simulink model "DblLaneChange_nn"  (R2018a)
settings: Solver=VariableStepAuto  StartTime=0.0  StopTime=10.0  RelTol=1e-3
libraries: neural x42
(part 2 of 2)

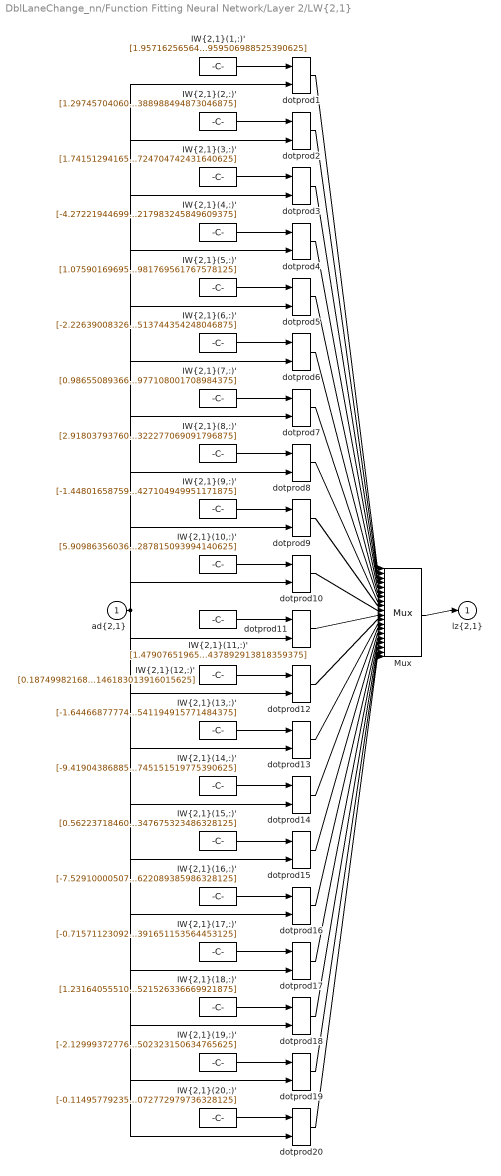
== system DblLaneChange_nn/Function Fitting Neural Network/Layer 2/LW{2,1} ==
  "ad{2,1}" : Inport  PortDimensions=15
      mask Display: e = 0.06;c1 = [120 230 180]/255;c2 = ([120 230 180]+0)/(256+128);c3 = ([120 230 180]+128)/(256+128);patch([0 1 1 0],[0 0 1 1],c1);patch([0 1 1 1-e 1-e 0+e],[0 0 1 1-e 0+e 0+e],c2);patch([0 0 1 1-e 0+e 0+e],[0 1 1 1-e 1-e 0+e],c3);plot([0 1 1 0 0],[0 0 1 1 0]);
  "IW{2,1}(1,:)'" : Constant  Value=[1.9571625656470332810243917265324853360652923583984375;3.8878561459758547158571673207916319370269775390625;2.015104111831793165521276023355312645435333251953125;-3.3420079123150543409792589955031871795654296875;-0.250819509672329743477092733883182518184185028076171875;0.6739952161544857656139129176153801381587982177734375;-1.3339737299760254796154868017765693366527557373046875;0.272342183832987583258500308147631585597991943359375;-0.04635129880112805189629199276168947108089923858642578125;-3.00793871482913033332806662656366825103759765625;0.251349256199478843232242297744960524141788482666015625;0.1750736907436108158453436089985189028084278106689453125;2.48237885981700845405839572777040302753448486328125;0.281589867390764025945060211597592569887638092041015625;-0.5513138093502016889857486603432334959506988525390625]
      mask Display: e = 0.06;c1 = [120 150 230]/255;c2 = ([120 150 230]+0)/383;c3 = ([120 150 230]+128)/383;patch([0 1 1 0],[0 0 1 1],c1);patch([0 1 1 1-e 1-e 0+e],[0 0 1 1-e 0+e 0+e],c2);patch([0 0 1 1-e 0+e 0+e],[0 1 1 1-e 1-e 0+e],c3);plot([0 1 1 0 0],[0 0 1 1 0]);disp('weights');
  "IW{2,1}(10,:)'" : Constant  Value=[5.90986356036200621844045599573291838169097900390625;-2.137684664328248107523222643067128956317901611328125;-3.226180872466682725274722542962990701198577880859375;2.398560219815558891554019282921217381954193115234375;-0.351261492817215692507915036912891082465648651123046875;1.756271886281308258759281670791096985340118408203125;-0.32097773012757924160354150444618426263332366943359375;2.0890044930821982660518187913112342357635498046875;-1.55820878601203549607134846155531704425811767578125;-0.399566441545824380110474294269806705415248870849609375;0.12749773005068154585472939288592897355556488037109375;0.0480334247417505133537218853234662674367427825927734375;0.0992931501305693575698541053498047403991222381591796875;-0.60598205258813242490845141219324432313442230224609375;-1.1258930863377900610799997593858279287815093994140625]
      mask Display: e = 0.06;c1 = [120 150 230]/255;c2 = ([120 150 230]+0)/383;c3 = ([120 150 230]+128)/383;patch([0 1 1 0],[0 0 1 1],c1);patch([0 1 1 1-e 1-e 0+e],[0 0 1 1-e 0+e 0+e],c2);patch([0 0 1 1-e 0+e 0+e],[0 1 1 1-e 1-e 0+e],c3);plot([0 1 1 0 0],[0 0 1 1 0]);disp('weights');
  "IW{2,1}(11,:)'" : Constant  Value=[1.479076519650180276954642977216280996799468994140625;-1.8264341661270770966751797459437511861324310302734375;-9.6450188180864966369654212030582129955291748046875;3.30452725241774469822075843694619834423065185546875;-1.062855642218289542455522678210400044918060302734375;2.373360663004012049981383825070224702358245849609375;-0.246008815611256370647907942839083261787891387939453125;-2.130860279171088667027333940495736896991729736328125;-2.00602923066542526697730863816104829311370849609375;-0.872186134418087011255238394369371235370635986328125;-6.687297405909703229553997516632080078125;1.364795272975333428888689013547264039516448974609375;-0.47158321560510074732519569806754589080810546875;-2.933715231286582625358505538315512239933013916015625;0.231501625263715649083451353362761437892913818359375]
      mask Display: e = 0.06;c1 = [120 150 230]/255;c2 = ([120 150 230]+0)/383;c3 = ([120 150 230]+128)/383;patch([0 1 1 0],[0 0 1 1],c1);patch([0 1 1 1-e 1-e 0+e],[0 0 1 1-e 0+e 0+e],c2);patch([0 0 1 1-e 0+e 0+e],[0 1 1 1-e 1-e 0+e],c3);plot([0 1 1 0 0],[0 0 1 1 0]);disp('weights');
  "IW{2,1}(12,:)'" : Constant  Value=[0.18749982168050538522408032804378308355808258056640625;-2.4186038350858876100346606108359992504119873046875;-0.54761726970257684765641670310287736356258392333984375;3.651368967093746586982661028741858899593353271484375;-0.70468135689368216478811746128485538065433502197265625;1.000020555024070834093663506791926920413970947265625;0.5891913103732548950830505418707616627216339111328125;4.00129895607543772939607151784002780914306640625;-0.460439945014462781447406314327963627874851226806640625;-0.6516061444199390262355109371128492057323455810546875;-0.2617198429841096629644425775040872395038604736328125;-0.8055231764580004227838117003557272255420684814453125;0.84533215292148700115149040357209742069244384765625;1.7135058705183412453010305398493073880672454833984375;0.214677382943929073721989198020310141146183013916015625]
      mask Display: e = 0.06;c1 = [120 150 230]/255;c2 = ([120 150 230]+0)/383;c3 = ([120 150 230]+128)/383;patch([0 1 1 0],[0 0 1 1],c1);patch([0 1 1 1-e 1-e 0+e],[0 0 1 1-e 0+e 0+e],c2);patch([0 0 1 1-e 0+e 0+e],[0 1 1 1-e 1-e 0+e],c3);plot([0 1 1 0 0],[0 0 1 1 0]);disp('weights');
  "IW{2,1}(13,:)'" : Constant  Value=[-1.6446687777437969391058913970482535660266876220703125;1.0892551228031204235691120629780925810337066650390625;-0.007684977593027149909976625252738813287578523159027099609375;1.86688177259719623179989866912364959716796875;-6.7794873490613216659994577639736235141754150390625;-0.418152455463235706023539250963949598371982574462890625;3.51712271643014862121390251559205353260040283203125;2.65031843964746460784454029635526239871978759765625;-5.3869854890003079361804338986985385417938232421875;-0.356673648884901439704009362685610540211200714111328125;-0.2295944669061752152483535382998525165021419525146484375;3.041459947956777210009704504045657813549041748046875;-1.628179163118948391542062381631694734096527099609375;-4.4714054694712874749029651866294443607330322265625;-2.741411485446989981795695712207816541194915771484375]
      mask Display: e = 0.06;c1 = [120 150 230]/255;c2 = ([120 150 230]+0)/383;c3 = ([120 150 230]+128)/383;patch([0 1 1 0],[0 0 1 1],c1);patch([0 1 1 1-e 1-e 0+e],[0 0 1 1-e 0+e 0+e],c2);patch([0 0 1 1-e 0+e 0+e],[0 1 1 1-e 1-e 0+e],c3);plot([0 1 1 0 0],[0 0 1 1 0]);disp('weights');
  "IW{2,1}(14,:)'" : Constant  Value=[-9.419043868851968426270104828290641307830810546875;2.114542513786489497107368151773698627948760986328125;6.6725367883884754149903528741560876369476318359375;2.461496243771723602122847296413965523242950439453125;2.012042505986927576344669432728551328182220458984375;-0.072474795090835986144384150975383818149566650390625;1.400146161122375332297451677732169628143310546875;-9.1458682032511955384279644931666553020477294921875;1.98598101723450337630083595286123454570770263671875;-4.45193123880581342888262952328659594058990478515625;2.451062197202027892473097381298430263996124267578125;-1.73850853038267150196816146490164101123809814453125;-2.06427192595482011938656796701252460479736328125;0.340728899158648401712667919127852655947208404541015625;0.67217341264327468142170118881040252745151519775390625]
      mask Display: e = 0.06;c1 = [120 150 230]/255;c2 = ([120 150 230]+0)/383;c3 = ([120 150 230]+128)/383;patch([0 1 1 0],[0 0 1 1],c1);patch([0 1 1 1-e 1-e 0+e],[0 0 1 1-e 0+e 0+e],c2);patch([0 0 1 1-e 0+e 0+e],[0 1 1 1-e 1-e 0+e],c3);plot([0 1 1 0 0],[0 0 1 1 0]);disp('weights');
  "IW{2,1}(15,:)'" : Constant  Value=[0.562237184609895468412332775187678635120391845703125;-0.9456920295664283937497884835465811192989349365234375;-0.6311954154726482357773420517332851886749267578125;3.275377370304279001089753364794887602329254150390625;0.329026190777529148334679121035151183605194091796875;-0.380998484745070420398604937872732989490032196044921875;-0.80017096636857443225920860641053877770900726318359375;1.73199083915180285231372181442566215991973876953125;-0.2276919016580762067381016322542564012110233306884765625;0.437211733838442084820741229123086668550968170166015625;-0.305821512121914995674387682811357080936431884765625;-1.38121314321437527183888960280455648899078369140625;0.844141753276321793464376241900026798248291015625;-3.458095739856301253922765681636519730091094970703125;1.2818508895183697848807469199527986347675323486328125]
      mask Display: e = 0.06;c1 = [120 150 230]/255;c2 = ([120 150 230]+0)/383;c3 = ([120 150 230]+128)/383;patch([0 1 1 0],[0 0 1 1],c1);patch([0 1 1 1-e 1-e 0+e],[0 0 1 1-e 0+e 0+e],c2);patch([0 0 1 1-e 0+e 0+e],[0 1 1 1-e 1-e 0+e],c3);plot([0 1 1 0 0],[0 0 1 1 0]);disp('weights');
  "IW{2,1}(16,:)'" : Constant  Value=[-7.52910000507232357591647087247110903263092041015625;2.34534452763346923376275299233384430408477783203125;2.634914709341771743567051089485175907611846923828125;-4.0266144720965275638491220888681709766387939453125;0.10282036662459941023239906598973902873694896697998046875;-1.3053476659419194216837922795093618333339691162109375;1.05964548882387976647123650764115154743194580078125;-2.941417987553542001677442385698668658733367919921875;0.82654152921551860000448641585535369813442230224609375;-0.2530410430159644175063249349477700889110565185546875;-0.1848911532609083530065419154198025353252887725830078125;6.47931547167705002010507087106816470623016357421875;-0.3942440277240584212137264330522157251834869384765625;4.01703752952216408544927617185749113559722900390625;1.886129375602820790192026834120042622089385986328125]
      mask Display: e = 0.06;c1 = [120 150 230]/255;c2 = ([120 150 230]+0)/383;c3 = ([120 150 230]+128)/383;patch([0 1 1 0],[0 0 1 1],c1);patch([0 1 1 1-e 1-e 0+e],[0 0 1 1-e 0+e 0+e],c2);patch([0 0 1 1-e 0+e 0+e],[0 1 1 1-e 1-e 0+e],c3);plot([0 1 1 0 0],[0 0 1 1 0]);disp('weights');
  "IW{2,1}(17,:)'" : Constant  Value=[-0.71571123092296196066541824620799161493778228759765625;-0.92777937570890145480007049627602100372314453125;10.8447708602443899650324965477921068668365478515625;1.4015710214659271581894017799641005694866180419921875;-0.10900237728617911958650665837922133505344390869140625;-3.064976767817614966560313405352644622325897216796875;1.3560856151338160913155661546625196933746337890625;0.88919198881820282753807305198279209434986114501953125;-0.76945576277128691078388555979472585022449493408203125;-4.0863512374290440476443109218962490558624267578125;3.79150612913527407243918787571601569652557373046875;1.2389275360579159457330433724564500153064727783203125;-3.55580501974170903878302851808257400989532470703125;-5.18367612230348751012343200272880494594573974609375;-2.193181481708041946632192775723524391651153564453125]
      mask Display: e = 0.06;c1 = [120 150 230]/255;c2 = ([120 150 230]+0)/383;c3 = ([120 150 230]+128)/383;patch([0 1 1 0],[0 0 1 1],c1);patch([0 1 1 1-e 1-e 0+e],[0 0 1 1-e 0+e 0+e],c2);patch([0 0 1 1-e 0+e 0+e],[0 1 1 1-e 1-e 0+e],c3);plot([0 1 1 0 0],[0 0 1 1 0]);disp('weights');
  "IW{2,1}(18,:)'" : Constant  Value=[1.2316405551040798815876087246579118072986602783203125;-2.102966577787353852357910000137053430080413818359375;2.058306439730734016535507180378772318363189697265625;1.5042854125219804473090334795415401458740234375;0.07703822108708051341618983087755623273551464080810546875;-1.449657194903263945917615274083800613880157470703125;2.148337007307501433928109690896235406398773193359375;-2.710709509179739740147851989604532718658447265625;0.60574839965657900631157417592476122081279754638671875;0.65562455406318942419119366604718379676342010498046875;-1.473787306106492334123458931571803987026214599609375;0.421496584121772766007296695534023456275463104248046875;-0.60631975751951083797308683642768301069736480712890625;-5.44685251089520594547366272308863699436187744140625;0.2398404687163100401647852777387015521526336669921875]
      mask Display: e = 0.06;c1 = [120 150 230]/255;c2 = ([120 150 230]+0)/383;c3 = ([120 150 230]+128)/383;patch([0 1 1 0],[0 0 1 1],c1);patch([0 1 1 1-e 1-e 0+e],[0 0 1 1-e 0+e 0+e],c2);patch([0 0 1 1-e 0+e 0+e],[0 1 1 1-e 1-e 0+e],c3);plot([0 1 1 0 0],[0 0 1 1 0]);disp('weights');
  "IW{2,1}(19,:)'" : Constant  Value=[-2.129993727764210031949687618180178105831146240234375;-1.1272107118748539988928314414806663990020751953125;-0.69156568999726408808470523581490851938724517822265625;0.73787856477719693248928933826391585171222686767578125;2.049753693423387534977564428118057548999786376953125;-3.34020954313206974717331831925548613071441650390625;3.015120023433614182550854820874519646167755126953125;-0.8669712765240202845262729169917292892932891845703125;-7.0815027415871920624113045050762593746185302734375;-4.7342133957354004536455249763093888759613037109375;-1.699728451389623362643988002673722803592681884765625;0.4915630144269445001015128582366742193698883056640625;0.663091540309036275857579312287271022796630859375;2.44407792172628379745447091409005224704742431640625;-0.0389738779121663603266512154732481576502323150634765625]
      mask Display: e = 0.06;c1 = [120 150 230]/255;c2 = ([120 150 230]+0)/383;c3 = ([120 150 230]+128)/383;patch([0 1 1 0],[0 0 1 1],c1);patch([0 1 1 1-e 1-e 0+e],[0 0 1 1-e 0+e 0+e],c2);patch([0 0 1 1-e 0+e 0+e],[0 1 1 1-e 1-e 0+e],c3);plot([0 1 1 0 0],[0 0 1 1 0]);disp('weights');
  "IW{2,1}(2,:)'" : Constant  Value=[1.2974570406068279826428124579251743853092193603515625;0.125214635833320098168286449435981921851634979248046875;1.311851249355715509636866045184433460235595703125;0.79447946068844255140817267601960338652133941650390625;2.814888454915816407009288013796322047710418701171875;-0.65002613849646484478483898783451877534389495849609375;0.31816623644248964719594141570269130170345306396484375;-4.21939598665019133250098093412816524505615234375;-1.2418665807473938667016000181320123374462127685546875;0.90699287127850503065218390474910847842693328857421875;-0.73688571392916613067569642225862480700016021728515625;-3.933466164463143233120945296832360327243804931640625;-1.0353306206281096546462094920570962131023406982421875;1.1599716225973069061438991411705501377582550048828125;0.78680595520741558601685028406791388988494873046875]
      mask Display: e = 0.06;c1 = [120 150 230]/255;c2 = ([120 150 230]+0)/383;c3 = ([120 150 230]+128)/383;patch([0 1 1 0],[0 0 1 1],c1);patch([0 1 1 1-e 1-e 0+e],[0 0 1 1-e 0+e 0+e],c2);patch([0 0 1 1-e 0+e 0+e],[0 1 1 1-e 1-e 0+e],c3);plot([0 1 1 0 0],[0 0 1 1 0]);disp('weights');
  "IW{2,1}(20,:)'" : Constant  Value=[-0.1149577923562907499910323849690030328929424285888671875;3.49330095989750599727585722575895488262176513671875;2.19885314886025273750647102133370935916900634765625;-0.2651349581561339707747038119123317301273345947265625;1.13861957041805705870274323388002812862396240234375;0.8131303347112022184006718816817738115787506103515625;-0.9470707754184870541536156451911665499210357666015625;-2.198780912367476414459588340832851827144622802734375;-1.294167608085416087959629294346086680889129638671875;1.2105212187917084865063088727765716612339019775390625;-1.0764523265034167121001473788055591285228729248046875;-2.26989440626234095788049671682529151439666748046875;0.037344458215924518362793804726607049815356731414794921875;0.477151102120123737915236006301711313426494598388671875;0.355409142713680126224318200911511667072772979736328125]
      mask Display: e = 0.06;c1 = [120 150 230]/255;c2 = ([120 150 230]+0)/383;c3 = ([120 150 230]+128)/383;patch([0 1 1 0],[0 0 1 1],c1);patch([0 1 1 1-e 1-e 0+e],[0 0 1 1-e 0+e 0+e],c2);patch([0 0 1 1-e 0+e 0+e],[0 1 1 1-e 1-e 0+e],c3);plot([0 1 1 0 0],[0 0 1 1 0]);disp('weights');
  "IW{2,1}(3,:)'" : Constant  Value=[1.7415129416524244287955980325932614505290985107421875;4.60958769398082690571527564316056668758392333984375;1.853953325328213441736124877934344112873077392578125;-2.29169405563924488689053760026581585407257080078125;0.64410752453107156245692976881400682032108306884765625;-0.420812285627358395601049778633750975131988525390625;-0.1909525372905495899100714041196624748408794403076171875;-0.784172476643829607922953073284588754177093505859375;2.125282454412551036426748396479524672031402587890625;0.1907080131010278345460307036773883737623691558837890625;0.109625387283181108255547542285057716071605682373046875;-3.505620102081777655911309921066276729106903076171875;-0.03136599554879802853601944434558390639722347259521484375;-2.232858007504352482186504857963882386684417724609375;-0.47777926155416994280500375680276192724704742431640625]
      mask Display: e = 0.06;c1 = [120 150 230]/255;c2 = ([120 150 230]+0)/383;c3 = ([120 150 230]+128)/383;patch([0 1 1 0],[0 0 1 1],c1);patch([0 1 1 1-e 1-e 0+e],[0 0 1 1-e 0+e 0+e],c2);patch([0 0 1 1-e 0+e 0+e],[0 1 1 1-e 1-e 0+e],c3);plot([0 1 1 0 0],[0 0 1 1 0]);disp('weights');
  "IW{2,1}(4,:)'" : Constant  Value=[-4.2722194469990757426103300531394779682159423828125;12.1359268792165782002712148823775351047515869140625;25.62472900977618195383911370299756526947021484375;2.7555733226685266146205322002060711383819580078125;3.490286334781497412649287070962600409984588623046875;-0.10529579464098215435541305851074866950511932373046875;-4.142639466636097722584963776171207427978515625;-2.08334429948006327748544208589009940624237060546875;6.00228296822584894698593416251242160797119140625;-2.08162749754345810515587800182402133941650390625;16.386586981025402565137483179569244384765625;-2.183350057131614452288204120122827589511871337890625;-9.718174177731981444594566710293292999267578125;0.053049440768477840180139537551440298557281494140625;-1.3102285593647200467870561624295078217983245849609375]
      mask Display: e = 0.06;c1 = [120 150 230]/255;c2 = ([120 150 230]+0)/383;c3 = ([120 150 230]+128)/383;patch([0 1 1 0],[0 0 1 1],c1);patch([0 1 1 1-e 1-e 0+e],[0 0 1 1-e 0+e 0+e],c2);patch([0 0 1 1-e 0+e 0+e],[0 1 1 1-e 1-e 0+e],c3);plot([0 1 1 0 0],[0 0 1 1 0]);disp('weights');
  "IW{2,1}(5,:)'" : Constant  Value=[1.075901696950349872849983512423932552337646484375;-0.85654332659910126235303096109419129788875579833984375;2.3929012059066661066708547878079116344451904296875;-2.3067434710526750762937808758579194545745849609375;-2.510749704465401688224801546311937272548675537109375;3.32161347428343400878247848595492541790008544921875;-1.175453029695316065073029676568694412708282470703125;-1.290711021437697780811504344455897808074951171875;0.945242250920026005900353993638418614864349365234375;4.1259010747603550584017284563742578029632568359375;-3.4282086004042948701453497051261365413665771484375;-1.49349992078351068158781345118768513202667236328125;1.9574683298787702856458281530649401247501373291015625;0.74543647882154961958889316520071588456630706787109375;1.80109180790346545819602397386915981769561767578125]
      mask Display: e = 0.06;c1 = [120 150 230]/255;c2 = ([120 150 230]+0)/383;c3 = ([120 150 230]+128)/383;patch([0 1 1 0],[0 0 1 1],c1);patch([0 1 1 1-e 1-e 0+e],[0 0 1 1-e 0+e 0+e],c2);patch([0 0 1 1-e 0+e 0+e],[0 1 1 1-e 1-e 0+e],c3);plot([0 1 1 0 0],[0 0 1 1 0]);disp('weights');
  "IW{2,1}(6,:)'" : Constant  Value=[-2.2263900832626379866496790782548487186431884765625;1.13140963270349370617395834415219724178314208984375;-1.1152718875630813766264282094198279082775115966796875;2.9638683900000462045909443986602127552032470703125;-0.119020542071015811291800901017268188297748565673828125;0.89580900077017833194048535006004385650157928466796875;0.89086444994895785942645716204424388706684112548828125;2.55474733870291981219224908272735774517059326171875;0.2169307183781970793656768137225299142301082611083984375;-1.0705850496691204920551854229415766894817352294921875;-0.2086614854452577827448322977943462319672107696533203125;3.9627646343637454862118829623796045780181884765625;1.2081351444333849887158294222899712622165679931640625;3.595934259547820754931990450131706893444061279296875;0.69768729317174216220109883579425513744354248046875]
      mask Display: e = 0.06;c1 = [120 150 230]/255;c2 = ([120 150 230]+0)/383;c3 = ([120 150 230]+128)/383;patch([0 1 1 0],[0 0 1 1],c1);patch([0 1 1 1-e 1-e 0+e],[0 0 1 1-e 0+e 0+e],c2);patch([0 0 1 1-e 0+e 0+e],[0 1 1 1-e 1-e 0+e],c3);plot([0 1 1 0 0],[0 0 1 1 0]);disp('weights');
  "IW{2,1}(7,:)'" : Constant  Value=[0.98655089366556480978687204697052948176860809326171875;2.1074232656800422347487256047315895557403564453125;-0.58570887409710092885717358512920327484607696533203125;0.48233336801888448963637756605749018490314483642578125;0.09963593409410780032953169893517042510211467742919921875;-0.46646130605211599817749856811133213341236114501953125;0.5093470115656264507464356938726268708705902099609375;0.794409715381384717858281874214299023151397705078125;1.988294947404373846921998847392387688159942626953125;-0.002675882203754468245671116477524265064857900142669677734375;-0.372645169229664563470549865087377838790416717529296875;-0.465779993386511048658604750016820617020130157470703125;0.5158318737046130308954161591827869415283203125;0.320477121396944786280158723457134328782558441162109375;0.11922148986793366931546955811427324078977108001708984375]
      mask Display: e = 0.06;c1 = [120 150 230]/255;c2 = ([120 150 230]+0)/383;c3 = ([120 150 230]+128)/383;patch([0 1 1 0],[0 0 1 1],c1);patch([0 1 1 1-e 1-e 0+e],[0 0 1 1-e 0+e 0+e],c2);patch([0 0 1 1-e 0+e 0+e],[0 1 1 1-e 1-e 0+e],c3);plot([0 1 1 0 0],[0 0 1 1 0]);disp('weights');
  "IW{2,1}(8,:)'" : Constant  Value=[2.918037937604385234635628876276314258575439453125;0.94424412902173404660288724699057638645172119140625;-0.2308796501149148749920669843049836345016956329345703125;-0.5007912878569114045745891417027451097965240478515625;7.38580232235594547063328718650154769420623779296875;1.148002415199903314402263276861049234867095947265625;-2.501848844515395686727288193651475012302398681640625;-1.0255996771174886728061892426921986043453216552734375;2.4956843839866085232870318577624857425689697265625;-1.8420465154428089515903366191196255385875701904296875;-0.5092823515801596645502513638348318636417388916015625;-1.5218477171204740638899011173634789884090423583984375;-0.6844739356845443989385557870264165103435516357421875;2.099767731690322047910512992530129849910736083984375;3.210608297261831278746058160322718322277069091796875]
      mask Display: e = 0.06;c1 = [120 150 230]/255;c2 = ([120 150 230]+0)/383;c3 = ([120 150 230]+128)/383;patch([0 1 1 0],[0 0 1 1],c1);patch([0 1 1 1-e 1-e 0+e],[0 0 1 1-e 0+e 0+e],c2);patch([0 0 1 1-e 0+e 0+e],[0 1 1 1-e 1-e 0+e],c3);plot([0 1 1 0 0],[0 0 1 1 0]);disp('weights');
  "IW{2,1}(9,:)'" : Constant  Value=[-1.4480165875975588019031192743568681180477142333984375;-3.23195010974846841378393946797586977481842041015625;-1.7682767350317025734085518706706352531909942626953125;2.702804363845552781953074372722767293453216552734375;-1.9772495347968772616553678744821809232234954833984375;2.048857644404706856988696017651818692684173583984375;1.01523318616815938497666138573549687862396240234375;-3.83537556144572366889633485698141157627105712890625;-0.4756332520795110152533879954717122018337249755859375;1.7277037976748832459605864642071537673473358154296875;0.10589567856046207261488945050587062723934650421142578125;2.186685152170862789233751755091361701488494873046875;-1.5394951106473524493623017406207509338855743408203125;-0.113300141138904797433184512556181289255619049072265625;-0.384121670028321815504313008204917423427104949951171875]
      mask Display: e = 0.06;c1 = [120 150 230]/255;c2 = ([120 150 230]+0)/383;c3 = ([120 150 230]+128)/383;patch([0 1 1 0],[0 0 1 1],c1);patch([0 1 1 1-e 1-e 0+e],[0 0 1 1-e 0+e 0+e],c2);patch([0 0 1 1-e 0+e 0+e],[0 1 1 1-e 1-e 0+e],c3);plot([0 1 1 0 0],[0 0 1 1 0]);disp('weights');
  Mux : Mux  Inputs=20
      mask Display: e = 0.06;c1 = [120 150 230]/255;c2 = ([120 150 230]+0)/383;c3 = ([120 150 230]+128)/383;patch([0 1 1 0],[0 0 1 1],c1);patch([0 1 1 1-e 1-e 0+e],[0 0 1 1-e 0+e 0+e],c2);patch([0 0 1 1-e 0+e 0+e],[0 1 1 1-e 1-e 0+e],c3);plot([0 1 1 0 0],[0 0 1 1 0]);disp('Mux');
  dotprod{1..20} (20 alike) : neural/Weight Functions/dotprod
  "lz{2,1}" : Outport
      mask Display: e = 0.06;c1 = [120 230 180]/255;c2 = ([120 230 180]+0)/(256+128);c3 = ([120 230 180]+128)/(256+128);patch([0 1 1 0],[0 0 1 1],c1);patch([0 1 1 1-e 1-e 0+e],[0 0 1 1-e 0+e 0+e],c2);patch([0 0 1 1-e 0+e 0+e],[0 1 1 1-e 1-e 0+e],c3);plot([0 1 1 0 0],[0 0 1 1 0]);
  wires:
  "IW{2,1}(1,:)'"/1 -> dotprod1/1
  "ad{2,1}"/1 -> dotprod1/2, dotprod2/2, dotprod3/2, dotprod4/2, dotprod5/2, dotprod6/2, dotprod7/2, dotprod8/2, dotprod9/2, dotprod10/2, dotprod11/2, dotprod12/2, dotprod13/2, dotprod14/2, dotprod15/2, dotprod16/2, dotprod17/2, dotprod18/2, dotprod19/2, dotprod20/2
  dotprod1/1 -> Mux/1
  "IW{2,1}(2,:)'"/1 -> dotprod2/1
  dotprod2/1 -> Mux/2
  "IW{2,1}(3,:)'"/1 -> dotprod3/1
  dotprod3/1 -> Mux/3
  "IW{2,1}(4,:)'"/1 -> dotprod4/1
  dotprod4/1 -> Mux/4
  "IW{2,1}(5,:)'"/1 -> dotprod5/1
  dotprod5/1 -> Mux/5
  "IW{2,1}(6,:)'"/1 -> dotprod6/1
  dotprod6/1 -> Mux/6
  "IW{2,1}(7,:)'"/1 -> dotprod7/1
  dotprod7/1 -> Mux/7
  "IW{2,1}(8,:)'"/1 -> dotprod8/1
  dotprod8/1 -> Mux/8
  "IW{2,1}(9,:)'"/1 -> dotprod9/1
  dotprod9/1 -> Mux/9
  "IW{2,1}(10,:)'"/1 -> dotprod10/1
  dotprod10/1 -> Mux/10
  "IW{2,1}(11,:)'"/1 -> dotprod11/1
  dotprod11/1 -> Mux/11
  "IW{2,1}(12,:)'"/1 -> dotprod12/1
  dotprod12/1 -> Mux/12
  "IW{2,1}(13,:)'"/1 -> dotprod13/1
  dotprod13/1 -> Mux/13
  "IW{2,1}(14,:)'"/1 -> dotprod14/1
  dotprod14/1 -> Mux/14
  "IW{2,1}(15,:)'"/1 -> dotprod15/1
  dotprod15/1 -> Mux/15
  "IW{2,1}(16,:)'"/1 -> dotprod16/1
  dotprod16/1 -> Mux/16
  "IW{2,1}(17,:)'"/1 -> dotprod17/1
  dotprod17/1 -> Mux/17
  "IW{2,1}(18,:)'"/1 -> dotprod18/1
  dotprod18/1 -> Mux/18
  "IW{2,1}(19,:)'"/1 -> dotprod19/1
  dotprod19/1 -> Mux/19
  "IW{2,1}(20,:)'"/1 -> dotprod20/1
  dotprod20/1 -> Mux/20
  Mux/1 -> "lz{2,1}"/1

== system DblLaneChange_nn/Function Fitting Neural Network/Layer 3/Delays 1 ==
  "p{3}" : Inport  PortDimensions=20
      mask Display: e = 0.06;c1 = [120 230 180]/255;c2 = ([120 230 180]+0)/(256+128);c3 = ([120 230 180]+128)/(256+128);patch([0 1 1 0],[0 0 1 1],c1);patch([0 1 1 1-e 1-e 0+e],[0 0 1 1-e 0+e 0+e],c2);patch([0 0 1 1-e 0+e 0+e],[0 1 1 1-e 1-e 0+e],c3);plot([0 1 1 0 0],[0 0 1 1 0]);
  mux : Mux  Inputs=1
      mask Display: e = 0.06;c1 = [120 150 230]/255;c2 = ([120 150 230]+0)/383;c3 = ([120 150 230]+128)/383;patch([0 1 1 0],[0 0 1 1],c1);patch([0 1 1 1-e 1-e 0+e],[0 0 1 1-e 0+e 0+e],c2);patch([0 0 1 1-e 0+e 0+e],[0 1 1 1-e 1-e 0+e],c3);plot([0 1 1 0 0],[0 0 1 1 0]);disp('Mux')
  "pd{3,2}" : Outport
      mask Display: e = 0.06;c1 = [120 230 180]/255;c2 = ([120 230 180]+0)/(256+128);c3 = ([120 230 180]+128)/(256+128);patch([0 1 1 0],[0 0 1 1],c1);patch([0 1 1 1-e 1-e 0+e],[0 0 1 1-e 0+e 0+e],c2);patch([0 0 1 1-e 0+e 0+e],[0 1 1 1-e 1-e 0+e],c3);plot([0 1 1 0 0],[0 0 1 1 0]);
  wires:
  "p{3}"/1 -> mux/1
  mux/1 -> "pd{3,2}"/1

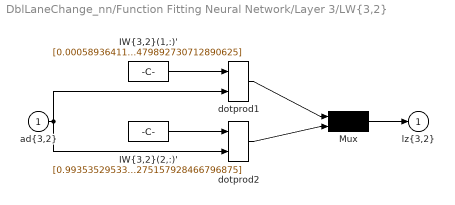
== system DblLaneChange_nn/Function Fitting Neural Network/Layer 3/LW{3,2} ==
  "ad{3,2}" : Inport  PortDimensions=20
      mask Display: e = 0.06;c1 = [120 230 180]/255;c2 = ([120 230 180]+0)/(256+128);c3 = ([120 230 180]+128)/(256+128);patch([0 1 1 0],[0 0 1 1],c1);patch([0 1 1 1-e 1-e 0+e],[0 0 1 1-e 0+e 0+e],c2);patch([0 0 1 1-e 0+e 0+e],[0 1 1 1-e 1-e 0+e],c3);plot([0 1 1 0 0],[0 0 1 1 0]);
  "IW{3,2}(1,:)'" : Constant  Value=[0.000589364117257014960386818369642014658893458545207977294921875;-1.70260737844308618349487005616538226604461669921875;-0.00029059056908142810726758398232050240039825439453125;-0.01216922302510307918321785791704314760863780975341796875;-0.000624817629691897208181472489485486221383325755596160888671875;-0.00085032860068717428490836507393169085844419896602630615234375;0.0003822919846798063236992248903334257192909717559814453125;3.8493742303641464985730635817162692546844482421875;0.0004286738740272564608668748320496888482011854648590087890625;-0.000717885808950110486208184834566736753913573920726776123046875;0.00033933201471113283442804231526679359376430511474609375;0.000594866322824000163561886100893616458051837980747222900390625;3.56039426454455831816403588163666427135467529296875;0.0003417524334987203358561524968450839878642000257968902587890625;-0.0002453138845937070824758385878539002078468911349773406982421875;-0.0002456227076207077712234616573283574325614608824253082275390625;-0.00079863942791508928976951242617587922723032534122467041015625;-0.000681822592969342903580776127370199901633895933628082275390625;2.938691678686937801940302905645552300484268926084041595458984375e-06;-1.6810547388690972869795814403914846479892730712890625]
      mask Display: e = 0.06;c1 = [120 150 230]/255;c2 = ([120 150 230]+0)/383;c3 = ([120 150 230]+128)/383;patch([0 1 1 0],[0 0 1 1],c1);patch([0 1 1 1-e 1-e 0+e],[0 0 1 1-e 0+e 0+e],c2);patch([0 0 1 1-e 0+e 0+e],[0 1 1 1-e 1-e 0+e],c3);plot([0 1 1 0 0],[0 0 1 1 0]);disp('weights');
  "IW{3,2}(2,:)'" : Constant  Value=[0.993535295331150702935474328114651143550872802734375;-0.056379468659354330106747710260606254450976848602294921875;2.2843805947014157453622829052619636058807373046875;-7.6565555501590676357182019273750483989715576171875;8.7955189817050527523178971023298799991607666015625;1.01533994017491924211071818717755377292633056640625;-1.2515123663875471482498369368840940296649932861328125;-0.1300380475608818031663105330153484828770160675048828125;0.2586320336462133440136312856338918209075927734375;2.000984935186024049613706665695644915103912353515625;-0.381496020856946060906267348400433547794818878173828125;0.75939563541428378723452397025539539754390716552734375;-0.08771849521104436997465114700389676727354526519775390625;-0.2432661951257036048179571707805735059082508087158203125;1.7098306922096477844519313293858431279659271240234375;1.92427407107717574064054133486934006214141845703125;8.871140875579811790885287337005138397216796875;0.442878318889609212671842897179885767400264739990234375;0.70453481172960719103315341271809302270412445068359375;3.0270033892703889222275392967276275157928466796875]
      mask Display: e = 0.06;c1 = [120 150 230]/255;c2 = ([120 150 230]+0)/383;c3 = ([120 150 230]+128)/383;patch([0 1 1 0],[0 0 1 1],c1);patch([0 1 1 1-e 1-e 0+e],[0 0 1 1-e 0+e 0+e],c2);patch([0 0 1 1-e 0+e 0+e],[0 1 1 1-e 1-e 0+e],c3);plot([0 1 1 0 0],[0 0 1 1 0]);disp('weights');
  Mux : Mux  Inputs=2
      mask Display: e = 0.06;c1 = [120 150 230]/255;c2 = ([120 150 230]+0)/383;c3 = ([120 150 230]+128)/383;patch([0 1 1 0],[0 0 1 1],c1);patch([0 1 1 1-e 1-e 0+e],[0 0 1 1-e 0+e 0+e],c2);patch([0 0 1 1-e 0+e 0+e],[0 1 1 1-e 1-e 0+e],c3);plot([0 1 1 0 0],[0 0 1 1 0]);disp('Mux');
  dotprod1 : neural/Weight Functions/dotprod
  dotprod2 : neural/Weight Functions/dotprod
  "lz{3,2}" : Outport
      mask Display: e = 0.06;c1 = [120 230 180]/255;c2 = ([120 230 180]+0)/(256+128);c3 = ([120 230 180]+128)/(256+128);patch([0 1 1 0],[0 0 1 1],c1);patch([0 1 1 1-e 1-e 0+e],[0 0 1 1-e 0+e 0+e],c2);patch([0 0 1 1-e 0+e 0+e],[0 1 1 1-e 1-e 0+e],c3);plot([0 1 1 0 0],[0 0 1 1 0]);
  wires:
  "IW{3,2}(1,:)'"/1 -> dotprod1/1
  "ad{3,2}"/1 -> dotprod1/2, dotprod2/2
  dotprod1/1 -> Mux/1
  "IW{3,2}(2,:)'"/1 -> dotprod2/1
  dotprod2/1 -> Mux/2
  Mux/1 -> "lz{3,2}"/1
